simulink model "vtolsim"  (R2020a)
settings: Solver=ode45  StartTime=0.0  StopTime=50  RelTol=1e-3  EnableMultiTasking=on
InitFcn:
  | clear all
  | path(pathdef)
  | addpath('.')
  | simulation_parameters
  | wind_parameters
  | vtol_parameters
StartFcn:
  | clear all
  | path(pathdef)
  | addpath('.')
  | simulation_parameters
  | wind_parameters
  | vtol_parameters
values from neighbouring files (symbols this model uses):
  vtol = P    [forces_moments.m]
undefined symbols (not defined in the file or in its folder): drawAircraft, forces_moments, init_states, plane_states, plotvtolstatevariables, SIM, vtol_dynamics, WIND
libraries: simulink x4
settings Model: Creator=beard  LastModifiedBy=VTOL_HYD
settings DataIOCC: LimitDataPoints=on  SaveFormat=Array  SignalLoggingSaveFormat=ModelDataLogs  ReturnWorkspaceOutputs=off
settings OptimizationCC: ExpressionDepthLimit=2147483647  InitFltsAndDblsToZero=on  LifeSpan=inf
settings DebuggingCC: UnderspecifiedInitializationDetection=Classic  MergeDetectMultiDrivingBlocksExec=none  SolverPrmCheckMsg=warning  FcnCallInpInsideContextMsg=warning  StateNameClashWarn=warning  PregeneratedLibrarySubsystemCodeDiagnostic=none  SFUnexpectedBacktrackingDiag=warning  SFNoUnconditionalDefaultTransitionDiag=warning  SFExecutionAtInitializationDiag=none  ArithmeticOperatorsInVariantConditions=warning
settings HardwareCC: ProdBitPerPointer=32  ProdBitPerSizeT=32  ProdBitPerPtrDiffT=32  ProdLargestAtomicFloat=None  ProdIntDivRoundTo=Undefined  ProdEndianess=Unspecified  ProdWordSize=32  ProdHWDeviceType=32-bit Generic
settings ModelReferenceCC: PropagateSignalLabelsOutOfModel=off
settings SFSimCC: SimUseLocalCustomCode=off  CustomCodeUndefinedFunction=UseInterfaceOnly
settings RTWCC: RTWUseLocalCustomCode=off
settings CodeAppCC: StateflowObjectComments=on
settings GRTTargetCC: TargetLangStandard=C89/C90 (ANSI)  CombineOutputUpdateFcns=off  GRTInterface=on
settings ConfigComp: CovMetricSettings=dw  CovHtmlReporting=on  CovSaveCumulativeToWorkspaceVar=on  CovSaveSingleToWorkspaceVar=on  CovExternalEMLEnable=off  CovSFcnEnable=off

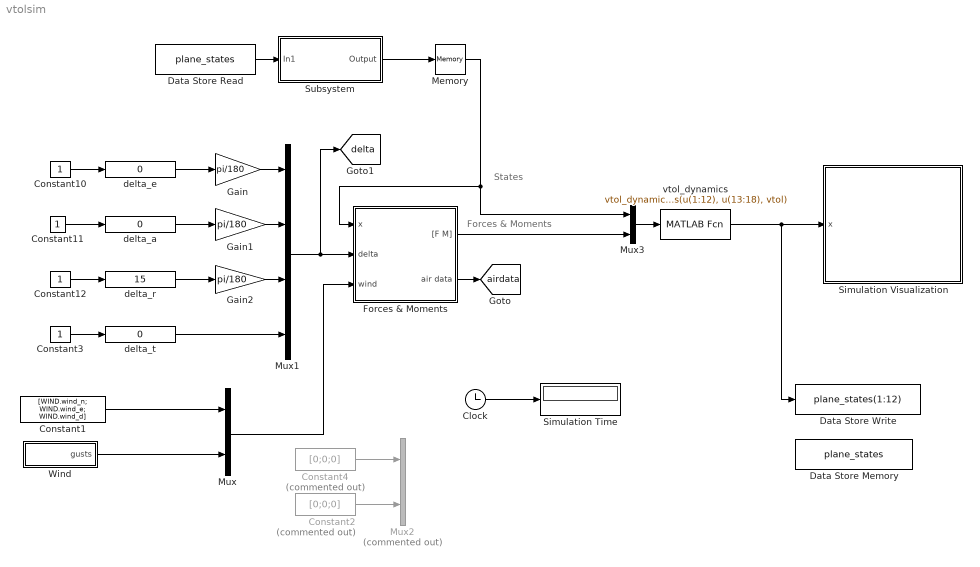
== system vtolsim ==
  note: Forces & Moments
  note: States
  Clock : Clock
  Constant1 : Constant  LoadFcn=|  InitFcn=|  StartFcn=|  Value=[WIND.wind_n; WIND.wind_e; WIND.wind_d]  SampleTime=SIM.ts_simulation
      | clear all
      | path(pathdef)
      | addpath('.')
      | simulation_parameters
      | wind_parameters
      | vtol_parameters
      | clear all
      | path(pathdef)
      | addpath('.')
      | simulation_parameters
      | wind_parameters
      | vtol_parameters
      | clear all
      | path(pathdef)
      | addpath('.')
      | simulation_parameters
      | wind_parameters
      | vtol_parameters
      settings: ContinueFcn=|
      | clear all
      | path(pathdef)
      | addpath('.')
      | simulation_parameters
      | wind_parameters
      | vtol_parameters
  Constant10 : Constant  LoadFcn=|  InitFcn=|  StartFcn=|  SampleTime=SIM.ts_simulation
      | clear all
      | path(pathdef)
      | addpath('.')
      | simulation_parameters
      | wind_parameters
      | vtol_parameters
      | clear all
      | path(pathdef)
      | addpath('.')
      | simulation_parameters
      | wind_parameters
      | vtol_parameters
      | clear all
      | path(pathdef)
      | addpath('.')
      | simulation_parameters
      | wind_parameters
      | vtol_parameters
      settings: ContinueFcn=|
      | clear all
      | path(pathdef)
      | addpath('.')
      | simulation_parameters
      | wind_parameters
      | vtol_parameters
  Constant11 : Constant  LoadFcn=|  InitFcn=|  StartFcn=|  SampleTime=SIM.ts_simulation
      | clear all
      | path(pathdef)
      | addpath('.')
      | simulation_parameters
      | wind_parameters
      | vtol_parameters
      | clear all
      | path(pathdef)
      | addpath('.')
      | simulation_parameters
      | wind_parameters
      | vtol_parameters
      | clear all
      | path(pathdef)
      | addpath('.')
      | simulation_parameters
      | wind_parameters
      | vtol_parameters
      settings: ContinueFcn=|
      | clear all
      | path(pathdef)
      | addpath('.')
      | simulation_parameters
      | wind_parameters
      | vtol_parameters
  Constant12 : Constant  LoadFcn=|  InitFcn=|  StartFcn=|  SampleTime=SIM.ts_simulation
      | clear all
      | path(pathdef)
      | addpath('.')
      | simulation_parameters
      | wind_parameters
      | vtol_parameters
      | clear all
      | path(pathdef)
      | addpath('.')
      | simulation_parameters
      | wind_parameters
      | vtol_parameters
      | clear all
      | path(pathdef)
      | addpath('.')
      | simulation_parameters
      | wind_parameters
      | vtol_parameters
      settings: ContinueFcn=|
      | clear all
      | path(pathdef)
      | addpath('.')
      | simulation_parameters
      | wind_parameters
      | vtol_parameters
  Constant2 : Constant  Commented=on  LoadFcn=|  InitFcn=|  StartFcn=|  Value=[0;0;0]  SampleTime=SIM.ts_simulation
      | clear all
      | path(pathdef)
      | addpath('.')
      | simulation_parameters
      | wind_parameters
      | vtol_parameters
      | clear all
      | path(pathdef)
      | addpath('.')
      | simulation_parameters
      | wind_parameters
      | vtol_parameters
      | clear all
      | path(pathdef)
      | addpath('.')
      | simulation_parameters
      | wind_parameters
      | vtol_parameters
      settings: ContinueFcn=|
      | clear all
      | path(pathdef)
      | addpath('.')
      | simulation_parameters
      | wind_parameters
      | vtol_parameters
  Constant3 : Constant  LoadFcn=|  InitFcn=|  StartFcn=|  SampleTime=SIM.ts_simulation
      | clear all
      | path(pathdef)
      | addpath('.')
      | simulation_parameters
      | wind_parameters
      | vtol_parameters
      | clear all
      | path(pathdef)
      | addpath('.')
      | simulation_parameters
      | wind_parameters
      | vtol_parameters
      | clear all
      | path(pathdef)
      | addpath('.')
      | simulation_parameters
      | wind_parameters
      | vtol_parameters
      settings: ContinueFcn=|
      | clear all
      | path(pathdef)
      | addpath('.')
      | simulation_parameters
      | wind_parameters
      | vtol_parameters
  Constant4 : Constant  Commented=on  LoadFcn=|  InitFcn=|  StartFcn=|  Value=[0;0;0]  SampleTime=SIM.ts_simulation
      | clear all
      | path(pathdef)
      | addpath('.')
      | simulation_parameters
      | wind_parameters
      | vtol_parameters
      | clear all
      | path(pathdef)
      | addpath('.')
      | simulation_parameters
      | wind_parameters
      | vtol_parameters
      | clear all
      | path(pathdef)
      | addpath('.')
      | simulation_parameters
      | wind_parameters
      | vtol_parameters
      settings: ContinueFcn=|
      | clear all
      | path(pathdef)
      | addpath('.')
      | simulation_parameters
      | wind_parameters
      | vtol_parameters
  Data Store Memory : DataStoreMemory  DataStoreName=plane_states  ReadBeforeWriteMsg=warning  WriteAfterWriteMsg=warning  WriteAfterReadMsg=warning  InitialValue=[0;0;0;0;0;0;0;0;0;0;0;0]  ShowAdditionalParam=off
  Data Store Read : DataStoreRead  DataStoreName=plane_states  SampleTime=SIM.ts_simulation
  Data Store Write : DataStoreWrite  DataStoreName=plane_states  SampleTime=SIM.ts_simulation  DataStoreElements=plane_states(1:12)
  Forces & Moments : Subsystem
  Gain : Gain  Gain=pi/180
  Gain1 : Gain  Gain=pi/180
  Gain2 : Gain  Gain=pi/180
  Memory : Memory
  Mux : Mux  Inputs=2
  Mux1 : Mux
  Mux2 : Mux  Commented=on  Inputs=2
  Mux3 : Mux  Inputs=2
  Simulation Time : Display
  Simulation Visualization : Subsystem
      mask Display: image(imread('../2_coord_frm/vtol.jpeg'))
  Subsystem : Subsystem  InitFcn=|
      | clear all
      | path(pathdef)
      | addpath('.')
  Wind : Subsystem  LoadFcn=|  InitFcn=|  StartFcn=|
      | clear all
      | path(pathdef)
      | addpath('.')
      | simulation_parameters
      | wind_parameters
      | vtol_parameters
      | clear all
      | path(pathdef)
      | addpath('.')
      | simulation_parameters
      | wind_parameters
      | vtol_parameters
      | clear all
      | path(pathdef)
      | addpath('.')
      | simulation_parameters
      | wind_parameters
      | vtol_parameters
  delta_a : simulink/Math Operations/Slider Gain  gain=0  low=-45  high=45
  delta_e : simulink/Math Operations/Slider Gain  gain=0  low=-45  high=45
  delta_r : simulink/Math Operations/Slider Gain  gain=15  low=-45  high=45
  delta_t : simulink/Math Operations/Slider Gain  gain=0  low=0  high=1
  vtol_dynamics : MATLABFcn  MATLABFcn=vtol_dynamics(u(1:12), u(13:18), vtol)  OutputDimensions=12
  tag scope: airdata=global, delta=global
  wires:
  Constant10/1 -> delta_e/1
  Constant11/1 -> delta_a/1
  Constant12/1 -> delta_r/1
  vtol_dynamics/1 -> Simulation Visualization/1(x), Data Store Write/1
  delta_r/1 -> Gain2/1
  delta_a/1 -> Gain1/1
  delta_e/1 -> Gain/1
  Constant3/1 -> delta_t/1
  delta_t/1 -> Mux1/4
  Mux1/1 -> [delta], Forces & Moments/2(delta)
  Forces & Moments/1("[F M]") -> Mux3/2
  Clock/1 -> Simulation Time/1
  Forces & Moments/2(air data) -> [airdata]
  Gain/1 -> Mux1/1
  Gain1/1 -> Mux1/2
  Gain2/1 -> Mux1/3
  Constant2/1 -> Mux2/2
  Data Store Read/1 -> Subsystem/1(In1)
  Mux3/1 -> vtol_dynamics/1
  Constant4/1 -> Mux2/1
  Mux/1 -> Forces & Moments/3(wind)
  Subsystem/1(Output) -> Memory/1
  Memory/1 -> Mux3/1, Forces & Moments/1(x)
  Wind/1(gusts) -> Mux/2
  Constant1/1 -> Mux/1

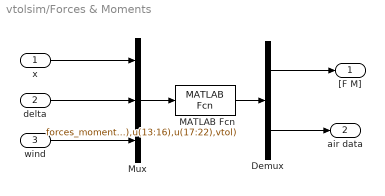
== system vtolsim/Forces & Moments ==
  x : Inport
  delta : Inport  Port=2
  wind : Inport  Port=3
  Demux : Demux  Outputs=[6;6]
  MATLAB Fcn : MATLABFcn  MATLABFcn=forces_moments(u(1:12),u(13:16),u(17:22),vtol)  OutputDimensions=12
  Mux : Mux  Inputs=3
  "[F M]" : Outport  VectorParamsAs1DForOutWhenUnconnected=off
  air data : Outport  Port=2  VectorParamsAs1DForOutWhenUnconnected=off
  wires:
  x/1 -> Mux/1
  delta/1 -> Mux/2
  wind/1 -> Mux/3
  MATLAB Fcn/1 -> Demux/1
  Demux/1 -> "[F M]"/1
  Mux/1 -> MATLAB Fcn/1
  Demux/2 -> air data/1

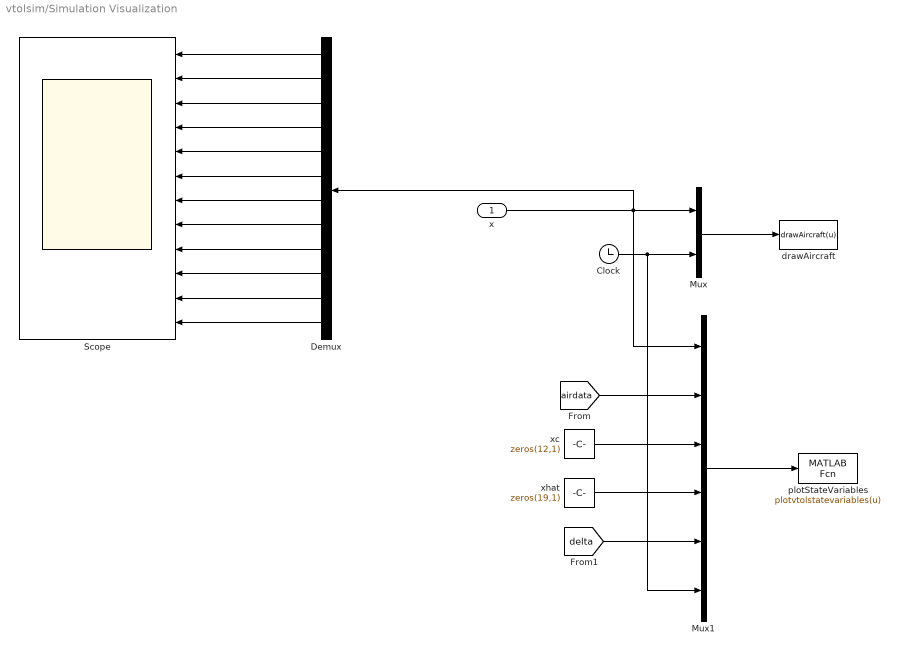
== system vtolsim/Simulation Visualization ==
  x : Inport
  Clock : Clock
  Demux : Demux  Outputs=12
  Mux : Mux  Inputs=2
  Mux1 : Mux  Inputs=6
  Scope : Scope  NumInputPorts=12
  drawAircraft : MATLABFcn  MATLABFcn=drawAircraft(u)  OutputDimensions=0  SampleTime=0.1
  plotStateVariables : MATLABFcn  MATLABFcn=plotvtolstatevariables(u)  OutputDimensions=0  SampleTime=0.01
  xc : Constant  Value=zeros(12,1)  SampleTime=SIM.ts_simulation
  xhat : Constant  Value=zeros(19,1)  SampleTime=SIM.ts_simulation
  wires:
  [airdata] -> Mux1/2
  [delta] -> Mux1/5
  xc/1 -> Mux1/3
  xhat/1 -> Mux1/4
  Mux1/1 -> plotStateVariables/1
  Clock/1 -> Mux1/6, Mux/2
  x/1 -> Demux/1, Mux1/1, Mux/1
  Mux/1 -> drawAircraft/1
  Demux/1 -> Scope/1
  Demux/2 -> Scope/2
  Demux/3 -> Scope/3
  Demux/4 -> Scope/4
  Demux/5 -> Scope/5
  Demux/6 -> Scope/6
  Demux/7 -> Scope/7
  Demux/8 -> Scope/8
  Demux/9 -> Scope/9
  Demux/10 -> Scope/10
  Demux/11 -> Scope/11
  Demux/12 -> Scope/12

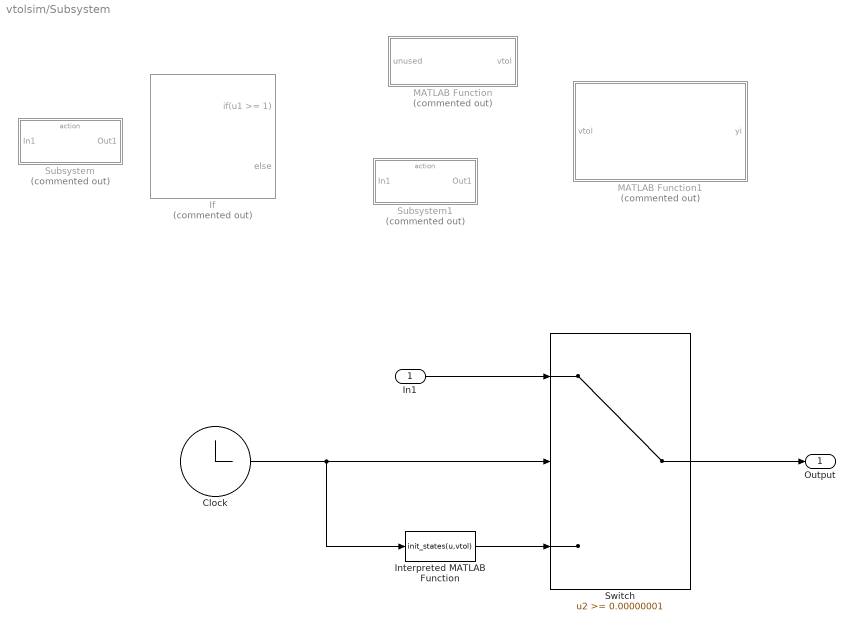
== system vtolsim/Subsystem ==
  In1 : Inport
  Clock : Clock
  If : If  Commented=on  IfExpression=u1 >= 1
  Interpreted MATLAB Function : MATLABFcn  MATLABFcn=init_states(u,vtol)  OutputDimensions=12
  MATLAB Function : MATLAB Function  Commented=on  TreatAsAtomicUnit=on
  MATLAB Function1 : MATLAB Function  Commented=on  InitFcn=|  TreatAsAtomicUnit=on
      | path(pathdef)
      | addpath('.')
  Subsystem : Subsystem  Commented=on
  Subsystem1 : Subsystem  Commented=on
  Switch : Switch  Threshold=0.00000001  ZeroCross=off
  Output : Outport  VectorParamsAs1DForOutWhenUnconnected=off
  wires:
  Switch/1 -> Output/1
  In1/1 -> Switch/1
  Interpreted MATLAB Function/1 -> Switch/3
  Clock/1 -> Interpreted MATLAB Function/1, Switch/2

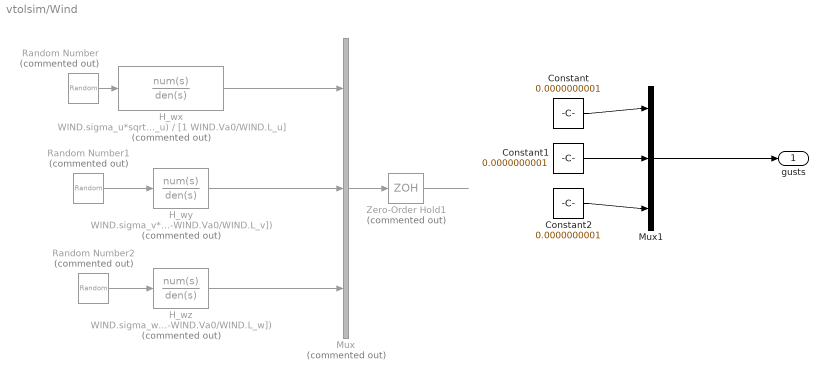
== system vtolsim/Wind ==
  Constant : Constant  Value=0.0000000001  SampleTime=SIM.ts_simulation
  Constant1 : Constant  Value=0.0000000001  SampleTime=SIM.ts_simulation
  Constant2 : Constant  Value=0.0000000001  SampleTime=SIM.ts_simulation
  H_wx : TransferFcn  Commented=on  Numerator=WIND.sigma_u*sqrt(2*WIND.Va0/WIND.L_u)  Denominator=[1 WIND.Va0/WIND.L_u]
  H_wy : TransferFcn  Commented=on  Numerator=WIND.sigma_v*sqrt(3*WIND.Va0/WIND.L_v)*[0, 1, WIND.Va0/sqrt(3)/WIND.L_v]  Denominator=poly([-WIND.Va0/WIND.L_v, -WIND.Va0/WIND.L_v])
  H_wz : TransferFcn  Commented=on  Numerator=WIND.sigma_w*sqrt(3*WIND.Va0/WIND.L_w)*[0, 1, WIND.Va0/sqrt(3)/WIND.L_w]  Denominator=poly([-WIND.Va0/WIND.L_w, -WIND.Va0/WIND.L_w])
  Mux : Mux  Commented=on  Inputs=3
  Mux1 : Mux  Inputs=3
  Random Number : RandomNumber  Commented=on  SampleTime=0
  Random Number1 : RandomNumber  Commented=on  SampleTime=0
  Random Number2 : RandomNumber  Commented=on  SampleTime=0
  Zero-Order Hold1 : ZeroOrderHold  Commented=on  SampleTime=SIM.ts_simulation
  gusts : Outport  VectorParamsAs1DForOutWhenUnconnected=off
  wires:
  H_wx/1 -> Mux/1
  Random Number/1 -> H_wx/1
  H_wy/1 -> Mux/2
  Random Number1/1 -> H_wy/1
  H_wz/1 -> Mux/3
  Random Number2/1 -> H_wz/1
  Mux1/1 -> gusts/1
  Constant/1 -> Mux1/1
  Constant2/1 -> Mux1/3
  Constant1/1 -> Mux1/2
  Zero-Order Hold1/1 -> ?
  Mux/1 -> Zero-Order Hold1/1

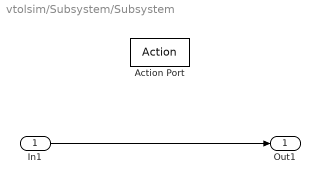
== system vtolsim/Subsystem/Subsystem ==
  In1 : Inport
  Action Port : ActionPort  InitializeStates=reset
  Out1 : Outport  VectorParamsAs1DForOutWhenUnconnected=off
  wires:
  In1/1 -> Out1/1

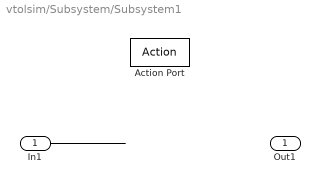
== system vtolsim/Subsystem/Subsystem1 ==
  In1 : Inport
  Action Port : ActionPort  InitializeStates=reset
  Out1 : Outport  VectorParamsAs1DForOutWhenUnconnected=off
  wires:
  In1/1 -> ?
  ? -> Out1/1

== matlab function vtolsim/Subsystem/MATLAB Function ==
  data: vtol output double; unused input
% initialize the VTOL viewer
function vtol = vtol_parameters(~)

    vtol.pn0    = 0;     % initial North position
	vtol.pe0    = 0;     % initial East position
	vtol.pd0    = 0;  % initial Down position (negative altitude)
	vtol.u0     = 0;     % initial velocity along body x-axis
	vtol.v0     = 0;     % initial velocity along body y-axis
	vtol.w0     = 0;     % initial velocity along body z-axis
	vtol.phi0   = 0;     % initial roll angle
	vtol.theta0 = 0;     % initial pitch angle
	vtol.psi0   = 0;     % initial yaw angle
% 	e = Euler2Quaternion(vtol.phi0,vtol.theta0,vtol.psi0);
% 	vtol.e0     = e(1);  % initial quaternion
% 	vtol.e1     = e(2);
% 	vtol.e2     = e(3);
% 	vtol.e3     = e(4);
	vtol.p0     = 0;     % initial body frame roll rate
	vtol.q0     = 0;     % initial body frame pitch rate
	vtol.r0     = 0;     % initial body frame yaw rate
    
	%physical parameters of airframe
	vtol.gravity = 9.81;
	vtol.mass = 13.5;
	vtol.Jx   = 0.8244;
	vtol.Jy   = 1.135;
	vtol.Jz   = 1.759;
	vtol.Jxz  = 0.1204;
	vtol.S_wing        = 0.55;
	vtol.b             = 2.90;
	vtol.c             = 0.19;
	vtol.S_prop        = 0.2027;
	vtol.rho           = 1.2682;
	vtol.e             = 0.9;
	vtol.AR            = vtol.b^2/vtol.S_wing;

	% Gamma parameters 
	vtol.Gamma  = vtol.Jx*vtol.Jz-vtol.Jxz^2;
	vtol.Gamma1 = (vtol.Jxz*(vtol.Jx-vtol.Jy+vtol.Jz))/vtol.Gamma;
	vtol.Gamma2 = (vtol.Jz*(vtol.Jz-vtol.Jy)+vtol.Jxz*vtol.Jxz)/vtol.Gamma;
	vtol.Gamma3 = vtol.Jz/vtol.Gamma;
	vtol.Gamma4 = vtol.Jxz/vtol.Gamma;
	vtol.Gamma5 = (vtol.Jz-vtol.Jx)/vtol.Jy;
	vtol.Gamma6 = vtol.Jxz/vtol.Jy;
	vtol.Gamma7 = (vtol.Jx*(vtol.Jx-vtol.Jy)+vtol.Jxz*vtol.Jxz)/vtol.Gamma;
	vtol.Gamma8 = vtol.Jx/vtol.Gamma;

	%%%%%%%%%%%%%%%%%%%%%%%%%%%%%%%%%
	% aerodynamic coefficients
	vtol.C_L_0         = 0.28;
	vtol.C_D_0         = 0.03;
	vtol.C_m_0         = -0.02338;
	vtol.C_L_alpha     = 3.45;
	vtol.C_D_alpha     = 0.30;
	vtol.C_m_alpha     = -0.38;
	vtol.C_L_q         = 0;
	vtol.C_D_q         = 0.0;
	vtol.C_m_q         = -3.6;
	vtol.C_L_delta_e   = -0.36;
	vtol.C_D_delta_e   = 0.0;
	vtol.C_m_delta_e   = -0.5;
	vtol.M             = 50;
	vtol.alpha0        = 0.4712;
	vtol.epsilon       = 0.16;
	vtol.C_D_p         = 0.0437;

	vtol.C_Y_0         = 0.0;
	vtol.C_ell_0       = 0.0;
	vtol.C_n_0         = 0.0;
	vtol.C_Y_beta      = -0.98;
	vtol.C_ell_beta    = -0.12;
	vtol.C_n_beta      = 0.25;
	vtol.C_Y_p         = 0.0;
	vtol.C_ell_p       = -0.26;
	vtol.C_n_p         = 0.022;
	vtol.C_Y_r         = 0.0;
	vtol.C_ell_r       = 0.14;
	vtol.C_n_r         = -0.35;
	vtol.C_Y_delta_a   = 0.0;
	vtol.C_ell_delta_a = 0.08;
	vtol.C_n_delta_a   = 0.06;
	vtol.C_Y_delta_r   = -0.17;
	vtol.C_ell_delta_r = 0.105;
	vtol.C_n_delta_r   = -0.032;

	% Parameters for propulsion thrust and torque models
	vtol.D_prop = 0.508;     % prop diameter in m

	% Motor parameters
	vtol.K_V = 145;                    % from datasheet RPM/V
	vtol.KQ = (1/vtol.K_V)*60/(2*pi);   % KQ in N-m/A, V-s/rad
	vtol.R_motor = 0.042;              % ohms
	vtol.i0 = 1.5;                     % no-load (zero-torque) current (A)

	% Inputs
	vtol.ncells = 12;
	vtol.V_max = 3.7*vtol.ncells;       % max voltage for specified number of battery cells

	% Coeffiecients from prop_data fit
	vtol.C_Q2 = -0.01664;
	vtol.C_Q1 = 0.004970;
	vtol.C_Q0 = 0.005230;

	vtol.C_T2 = -0.1079;
	vtol.C_T1 = -0.06044;
	vtol.C_T0 = 0.09357;

end

== matlab function vtolsim/Subsystem/MATLAB Function1 ==
  data: yi output; vtol input
function yi = init_states(vtol)
   yi = vtol;
end
